simulink model "pwm"  (R2013b)
settings: Solver=ode4  StartTime=0.0  StopTime=20  FixedStep=0.001  RelTol=1e-3
settings Model: Creator=Test  LastModifiedBy=Test

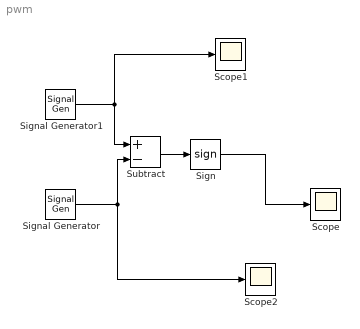
== system pwm ==
  Scope : Scope
      settings: TimeRange=20  YMin=-1  YMax=2
  Scope1 : Scope
  Scope2 : Scope
      settings: YMin=-1  YMax=1  SaveName=ScopeData2
  Sign : Signum
  Signal Generator : SignalGenerator  WaveForm=sawtooth  Frequency=12
  Signal Generator1 : SignalGenerator  Frequency=2  Units=rad/sec
  Subtract : Sum  Inputs=+-
  wires:
  Signal Generator1/1 -> Subtract/1, Scope1/1
  Signal Generator/1 -> Subtract/2, Scope2/1
  Subtract/1 -> Sign/1
  Sign/1 -> Scope/1
